simulink model "CoVM_SpdCoord"  (R2016b)
settings: configuration reference "CodeGenConfigSet" (kept outside this file)
values from neighbouring files (symbols this model uses):
  EPM_N_MAX = uint16(10000)    [init_CoVM_SpdCoord.m]
  EPM_N_ZERO = uint16(0)    [init_CoVM_SpdCoord.m]
settings Model: Creator=Administrator  LastModifiedBy=Administrator
settings ConfigSetRef: SourceLocation=Base Workspace

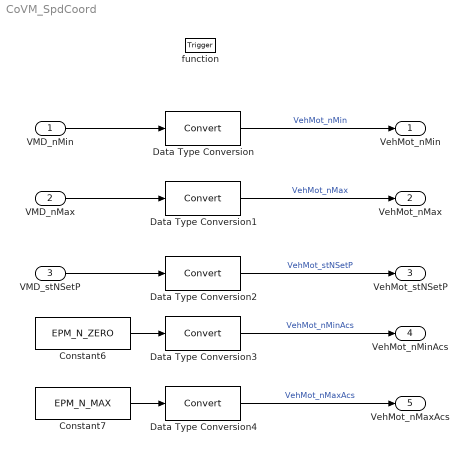
== system CoVM_SpdCoord ==
  VMD_nMin : Inport  Tag=rpm  Description=Minimum engine speed limitation after driving assistance coordination  OutMin=-12000  OutMax=12000  OutDataTypeStr=EngSpeed_rpm
  VMD_nMax : Inport  Tag=rpm  Description=Maximum engine speed limitation after driving assistance coordination  Port=2  OutMin=-12000  OutMax=12000  OutDataTypeStr=EngSpeed_rpm
  VMD_stNSetP : Inport  Description=Status of engine speed request after driving assistance coordination  Port=3  OutMin=0  OutMax=255  OutDataTypeStr=State_uint8
  function : TriggerPort  TriggerType=function-call  VariantControl=Variant
  Constant6 : Constant  Value=EPM_N_ZERO  OutDataTypeStr=EngSpeed_rpm
  Constant7 : Constant  Value=EPM_N_MAX  OutDataTypeStr=EngSpeed_rpm
  Data Type Conversion{,1..4} (5 alike) : DataTypeConversion
  VehMot_nMin : Outport  Tag=rpm  Description=Minimum engine speed for VehMot  OutMin=-12000  OutMax=12000  OutDataTypeStr=EngSpeed_rpm
  VehMot_nMax : Outport  Tag=rpm  Description=Maximum engine speed for VehMot  Port=2  OutMin=-12000  OutMax=12000  OutDataTypeStr=EngSpeed_rpm
  VehMot_stNSetP : Outport  Description=Status of engine speed request after driving assistance coordination  Port=3  OutMin=0  OutMax=255  OutDataTypeStr=State_uint8
  VehMot_nMinAcs : Outport  Tag=rpm  Description=Minimum engine speed demand by accessories of Vehicle Motion  Port=4  OutMin=-12000  OutMax=12000  OutDataTypeStr=EngSpeed_rpm
  VehMot_nMaxAcs : Outport  Tag=rpm  Description=Maximum engine speed demand by accessories of Vehicle Motion  Port=5  OutMin=-12000  OutMax=12000  OutDataTypeStr=EngSpeed_rpm
  wires:
  Data Type Conversion2/1 -> VehMot_stNSetP/1  "VehMot_stNSetP"
  Constant6/1 -> Data Type Conversion3/1
  Constant7/1 -> Data Type Conversion4/1
  VMD_nMax/1 -> Data Type Conversion1/1
  Data Type Conversion1/1 -> VehMot_nMax/1  "VehMot_nMax"
  Data Type Conversion/1 -> VehMot_nMin/1  "VehMot_nMin"
  VMD_stNSetP/1 -> Data Type Conversion2/1
  VMD_nMin/1 -> Data Type Conversion/1
  Data Type Conversion3/1 -> VehMot_nMinAcs/1  "VehMot_nMinAcs"
  Data Type Conversion4/1 -> VehMot_nMaxAcs/1  "VehMot_nMaxAcs"
